simulink model "PlatformModeManager"  (R2026a)
settings: Solver=FixedStepDiscrete  StopTime=10  FixedStep=0.1
model workspace (MAT data in the model file):
  soc_low = 0.4
  soc_safe_stop = 0.1
Description:
  | PROPOSED platform mode manager for rover_safety (SYS-SR-010). Generated by scripts/build_mode_manager.m.
settings Model: Creator=potlo  LastModifiedBy=potlo
settings DataIOCC: LoadExternalInput=on

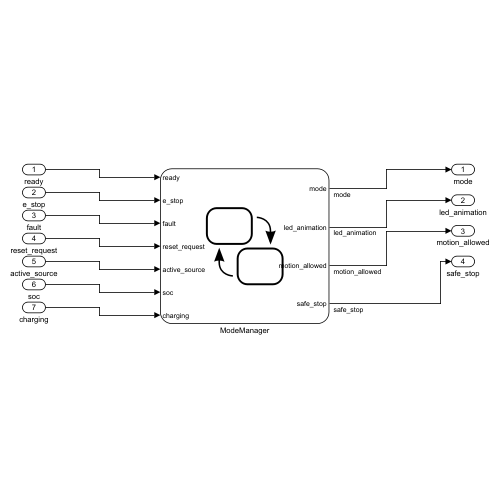
[thumbnail: Simulink's stored preview of the top-level diagram]
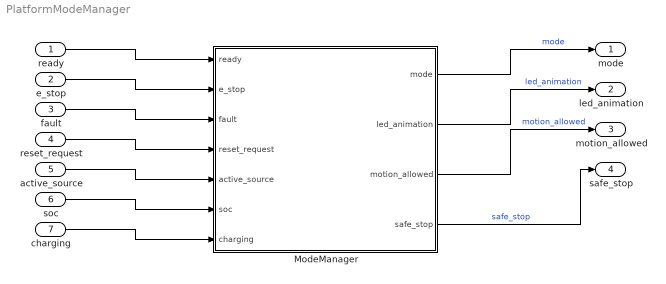
== system PlatformModeManager ==
  ready : Inport  Interpolate=off
  e_stop : Inport  Port=2  Interpolate=off
  fault : Inport  Port=3  Interpolate=off
  reset_request : Inport  Port=4  Interpolate=off
  active_source : Inport  Port=5  Interpolate=off
  soc : Inport  Port=6  Interpolate=off
  charging : Inport  Port=7  Interpolate=off
  ModeManager : Stateflow chart  TreatAsAtomicUnit=on
  mode : Outport
  led_animation : Outport  Port=2
  motion_allowed : Outport  Port=3
  safe_stop : Outport  Port=4
  wires:
  ready/1 -> ModeManager/1(ready)
  e_stop/1 -> ModeManager/2(e_stop)
  fault/1 -> ModeManager/3(fault)
  reset_request/1 -> ModeManager/4(reset_request)
  active_source/1 -> ModeManager/5(active_source)
  soc/1 -> ModeManager/6(soc)
  charging/1 -> ModeManager/7(charging)
  ModeManager/1(mode) -> mode/1  "mode"
  ModeManager/2(led_animation) -> led_animation/1  "led_animation"
  ModeManager/3(motion_allowed) -> motion_allowed/1  "motion_allowed"
  ModeManager/4(safe_stop) -> safe_stop/1  "safe_stop"

== stateflow chart PlatformModeManager/ModeManager ==
  settings: updateMethod=DISCRETE  sampleTime=0.1
  state Boot
    entry: mode = 0; led_animation = 255; motion_allowed = 0; safe_stop = 0;
  state EmergencyStop
    entry: mode = 4; led_animation = 0; motion_allowed = 0; safe_stop = 0;
  state Fault
    entry: mode = 5; led_animation = 2; motion_allowed = 0; safe_stop = 0;
  state Operational
    state Idle
      entry: mode = 1; led_animation = 1; motion_allowed = 1; safe_stop = 0;
    state Teleoperation
      entry: mode = 2; led_animation = 4; motion_allowed = 1; safe_stop = 0;
    state Autonomous
      entry: mode = 3; led_animation = 12; motion_allowed = 1; safe_stop = 0;
    (default) -> Idle
    Idle -> Teleoperation [order 1] : [active_source >= 1 && active_source <= 3]
    Teleoperation -> Autonomous [order 1] : [active_source == 4]
    Teleoperation -> Idle [order 2] : [active_source == 0]
    Autonomous -> Teleoperation [order 1] : [active_source >= 1 && active_source <= 3]
    Autonomous -> Idle [order 2] : [active_source == 0]
  state LowBattery
    state Warning
      entry: mode = 6; led_animation = 5; motion_allowed = 1; safe_stop = 0;
    state SafeStop
      entry: mode = 6; led_animation = 6; motion_allowed = 0; safe_stop = 1;
    (default) -> Warning
    Warning -> SafeStop : [soc < soc_safe_stop]
  (default) -> Boot
  Boot -> Operational [order 2] : [ready > 0.5]
  Boot -> EmergencyStop [order 1] : [ready > 0.5 && e_stop > 0.5]
  EmergencyStop -> Fault [order 1] : [e_stop < 0.5 && fault > 0.5]
  Fault -> EmergencyStop [order 1] : [e_stop > 0.5]
  Operational -> EmergencyStop [order 1] : [e_stop > 0.5]
  EmergencyStop -> Operational [order 2] : [e_stop < 0.5]
  LowBattery -> EmergencyStop [order 1] : [e_stop > 0.5]
  Operational -> Fault [order 2] : [fault > 0.5]
  Fault -> Operational [order 2] : [fault < 0.5 && reset_request > 0.5]
  LowBattery -> Fault [order 2] : [fault > 0.5]
  Idle -> Autonomous [order 2] : [active_source == 4]
  Operational -> LowBattery [order 3] : [soc < soc_low && charging < 0.5]
  LowBattery -> Operational [order 3] : [soc >= soc_low || charging > 0.5]
  data: ready input double; e_stop input double; fault input double; reset_request input double; active_source input double; soc input double; charging input double; mode output double; led_animation output double; motion_allowed output double; safe_stop output double; soc_low parameter; soc_safe_stop parameter
